simulink model "slAccelDemoWhyRebuild"  (Simulink 7.6)
settings: Solver=ode1  StartTime=0.0  StopTime=1  FixedStep=1  RelTol=1e-3
undefined symbols (not defined in the file or in its folder): clock
settings Model: Creator=The MathWorks Inc.  SimulationMode=accelerator  ExtModeAutoUpdateStatusClock=off
settings DataIOCC: SignalLoggingName=logsOut
settings OptimizationCC: BooleanDataType=off  InlineParams=on  InitFltsAndDblsToZero=on
settings DebuggingCC: SaveWithParameterizedLinksMsg=none  SignalResolutionControl=TryResolveAllWithWarning  SolverPrmCheckMsg=none  MultiTaskDSMMsg=warning  MultiTaskCondExecSysMsg=none
settings HardwareCC: TargetUnknown=on
settings RTWCC: IncludeERTFirstTime=on
settings GRTTargetCC: TargetFcnLib=ansi_tfl_tmw.mat

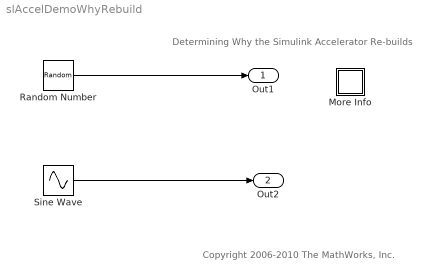
== system slAccelDemoWhyRebuild ==
  note: Determining Why the Simulink Accelerator Re-builds
  note: Copyright 2006-2010 The MathWorks, Inc.
  More Info : Subsystem
      settings: OpenFcn=showdemo('slAccelDemoWhyRebuild_script')
      mask Display: disp('?')
  Random Number : RandomNumber  Seed=floor((sum(clock)+rand)*10000)  SampleTime=0
  Sine Wave : Sin  SampleTime=0
  Out1 : Outport
  Out2 : Outport  Port=2
  wires:
  Sine Wave/1 -> Out2/1
  Random Number/1 -> Out1/1

== system slAccelDemoWhyRebuild/More Info ==
